simulink model "FD_example_2018b"  (R2018b)
settings: Solver=ode1  StartTime=0.0  StopTime=inf  FixedStep=1e-3  RelTol=1e-3
InitFcn:
  | plant = Dexmart_index;
  | plant_mdh = mdh_struct_to_matrix(plant.mdh_ori,1);
  | 
  | % init value for solver
  | q_init = zeros(plant.nj,1);
  | qD_init = zeros(plant.nj,1);
  | 
  | % parameters for passive properties
  | K_q = 1e1;% stiffness Nm/rad
  | q0_stiff = [0;pi/6;pi/4;pi/6];
  | D_q = 5; % Damping of joint
  | 
  | % parameter for controller
  | grv_comp_on = 0;
  | K_ctrl = 0;
  | D_ctrl = 0;
  | 
  | 
  | % desired x
  | 
  | x_desired = [rand(plant.nj,1);zeros(plant.nj,1)];
model workspace: external: MAT-File D:\repos\hand_modeling_toolbox\examples\hand_one\hand_one_model.mat (data not in the file)
values from neighbouring files (symbols this model uses):
  Dexmart_index = Finger('Index_Dexmart', 'type','R_RRRR', 'l_links',finger_index_dimension)    [create_Dexmart_index.m]
settings Model: Creator=ge26jow  LastModifiedBy=ge26jow
settings DataIOCC: ReturnWorkspaceOutputs=on
settings DebuggingCC: SFMachineParentedDataDiag=error

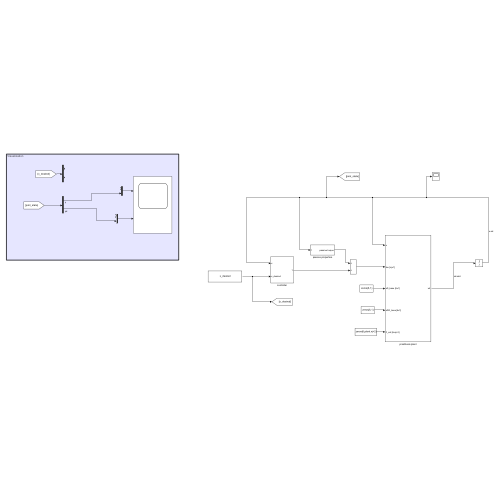
[thumbnail: Simulink's stored preview of the top-level diagram]
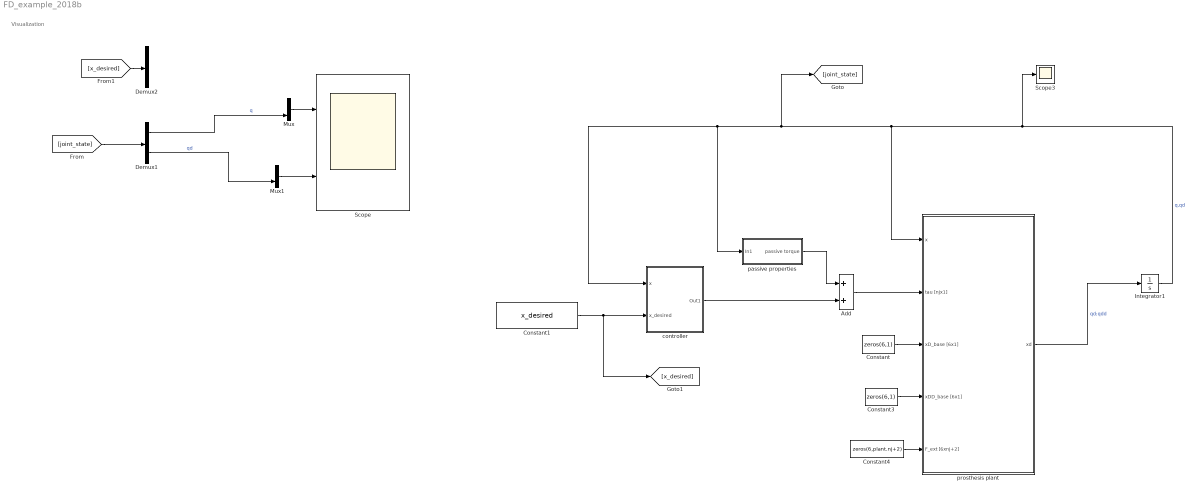
== system FD_example_2018b ==
  note: Visualization
  Add : Sum
  Constant : Constant  Value=zeros(6,1)
  Constant1 : Constant  Value=x_desired
  Constant3 : Constant  Value=zeros(6,1)
  Constant4 : Constant  Value=zeros(6,plant.nj+2)
  Demux1 : Demux  Outputs=[plant.nj,plant.nj]
  Demux2 : Demux  Outputs=[plant.nj,plant.nj]
  Integrator1 : Integrator  InitialCondition=[q_init;qD_init]  WrappedStateUpperValue=[pi,pi,pi,pi,1e4,1e4,1e4,1e4]  WrappedStateLowerValue=-[pi,pi,pi,pi,1e4,1e4,1e4,1e4]
  Mux : Mux  Inputs=2
  Mux1 : Mux  Inputs=2
  Scope : Scope  NumInputPorts=2
  Scope3 : Scope
  controller : Subsystem
  passive properties : Subsystem
  prosthesis plant : Subsystem
  wires:
  Add/1 -> prosthesis plant/2(tau [njx1])
  prosthesis plant/1(xd) -> Integrator1/1  "qd;qdd"
  Integrator1/1 -> [joint_state], controller/1(x), passive properties/1(In1), prosthesis plant/1(x), Scope3/1  "q,qd"
  Constant/1 -> prosthesis plant/3(xD_base [6x1])
  Constant3/1 -> prosthesis plant/4(xDD_base [6x1])
  Constant4/1 -> prosthesis plant/5(F_ext [6xnj+2])
  passive properties/1(passive torque) -> Add/1
  [joint_state] -> Demux1/1
  controller/1(Out1) -> Add/2
  Constant1/1 -> [x_desired], controller/2(x_desired)
  [x_desired] -> Demux2/1
  Demux1/1 -> Mux/2  "q"
  Mux/1 -> Scope/1
  Mux1/1 -> Scope/2
  Demux1/2 -> Mux1/2  "qd"

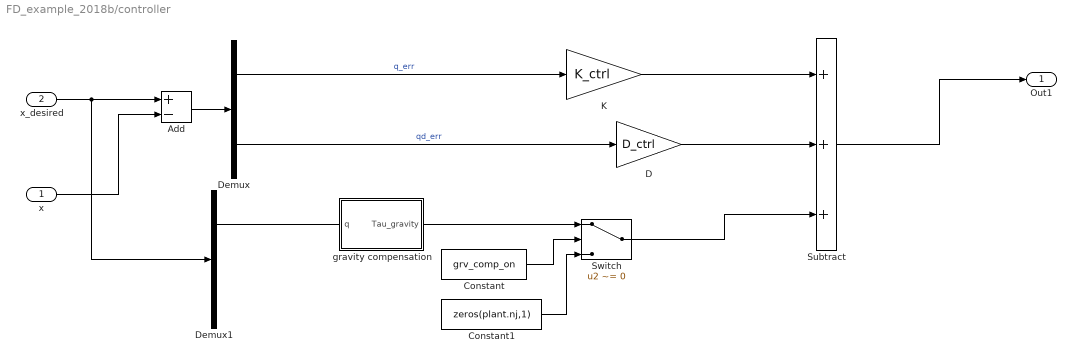
== system FD_example_2018b/controller ==
  x : Inport
  x_desired : Inport  Port=2
  Add : Sum  Inputs=+-
  Constant : Constant  Value=grv_comp_on
  Constant1 : Constant  Value=zeros(plant.nj,1)
  D : Gain  Gain=D_ctrl
  Demux : Demux  Outputs=[plant.nj,plant.nj]
  Demux1 : Demux  Outputs=[plant.nj,plant.nj]
  K : Gain  Gain=K_ctrl
  Subtract : Sum  Inputs=+++
  Switch : Switch  Criteria=u2 ~= 0
  gravity compensation : Subsystem
  Out1 : Outport
  wires:
  K/1 -> Subtract/1
  D/1 -> Subtract/2
  Subtract/1 -> Out1/1
  Demux/2 -> D/1  "qd_err"
  Demux/1 -> K/1  "q_err"
  Add/1 -> Demux/1
  x/1 -> Add/2
  x_desired/1 -> Demux1/1, Add/1
  Demux1/1 -> gravity compensation/1(q)
  Constant/1 -> Switch/2
  gravity compensation/1(Tau_gravity) -> Switch/1
  Switch/1 -> Subtract/3
  Constant1/1 -> Switch/3

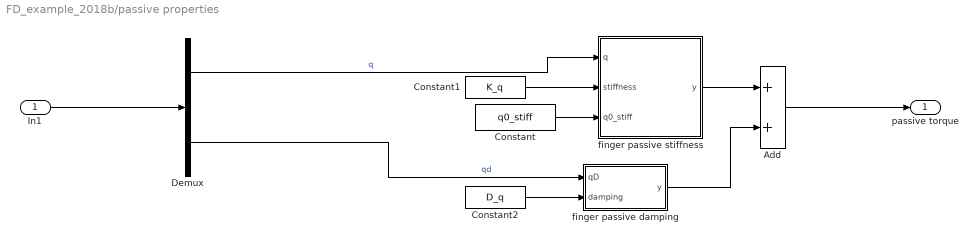
== system FD_example_2018b/passive properties ==
  In1 : Inport
  Add : Sum
  Constant : Constant  Value=q0_stiff
  Constant1 : Constant  Value=K_q
  Constant2 : Constant  Value=D_q
  Demux : Demux  Outputs=[plant.nj,plant.nj]
  finger passive damping : MATLAB Function  TreatAsAtomicUnit=on
  finger passive stiffness : MATLAB Function  TreatAsAtomicUnit=on
  passive torque : Outport
  wires:
  Constant2/1 -> finger passive damping/2(damping)
  finger passive damping/1(y) -> Add/2
  Demux/2 -> finger passive damping/1(qD)  "qd"
  Constant1/1 -> finger passive stiffness/2(stiffness)
  finger passive stiffness/1(y) -> Add/1
  Demux/1 -> finger passive stiffness/1(q)  "q"
  In1/1 -> Demux/1
  Constant/1 -> finger passive stiffness/3(q0_stiff)
  Add/1 -> passive torque/1

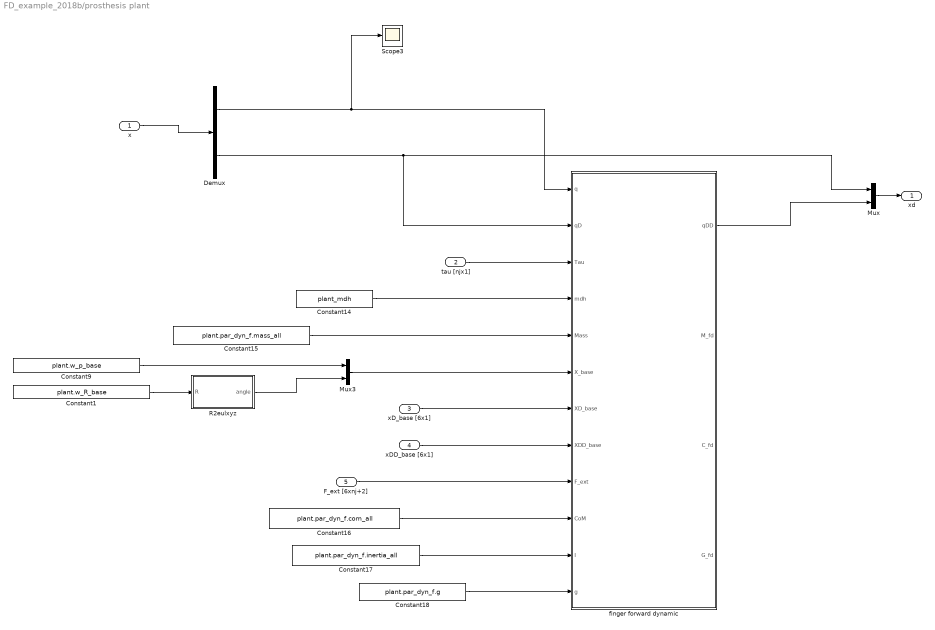
== system FD_example_2018b/prosthesis plant ==
  x : Inport
  tau [njx1] : Inport  Port=2
  xD_base [6x1] : Inport  Port=3
  xDD_base [6x1] : Inport  Port=4
  F_ext [6xnj+2] : Inport  Port=5
  Constant1 : Constant  Value=plant.w_R_base
  Constant14 : Constant  Value=plant_mdh
  Constant15 : Constant  Value=plant.par_dyn_f.mass_all
  Constant16 : Constant  Value=plant.par_dyn_f.com_all
  Constant17 : Constant  Value=plant.par_dyn_f.inertia_all
  Constant18 : Constant  Value=plant.par_dyn_f.g
  Constant9 : Constant  Value=plant.w_p_base
  Demux : Demux  Outputs=[plant.nj,plant.nj]
  Mux : Mux  Inputs=2
  Mux3 : Mux  Inputs=[3,3]
  R2eulxyz : MATLAB Function  TreatAsAtomicUnit=on
  Scope3 : Scope
  finger forward dynamic : MATLAB Function  TreatAsAtomicUnit=on
  xd : Outport
  wires:
  Constant18/1 -> finger forward dynamic/12(g)
  tau [njx1]/1 -> finger forward dynamic/3(Tau)
  Constant17/1 -> finger forward dynamic/11(I)
  finger forward dynamic/1(qDD) -> Mux/2
  Demux/2 -> finger forward dynamic/2(qD), Mux/1
  Mux3/1 -> finger forward dynamic/6(X_base)
  Constant14/1 -> finger forward dynamic/4(mdh)
  Demux/1 -> Scope3/1, finger forward dynamic/1(q)
  F_ext [6xnj+2]/1 -> finger forward dynamic/9(F_ext)
  Constant15/1 -> finger forward dynamic/5(Mass)
  Constant16/1 -> finger forward dynamic/10(CoM)
  Mux/1 -> xd/1
  Constant1/1 -> R2eulxyz/1(R)
  R2eulxyz/1(angle) -> Mux3/2
  Constant9/1 -> Mux3/1
  x/1 -> Demux/1
  xD_base [6x1]/1 -> finger forward dynamic/7(XD_base)
  xDD_base [6x1]/1 -> finger forward dynamic/8(XDD_base)

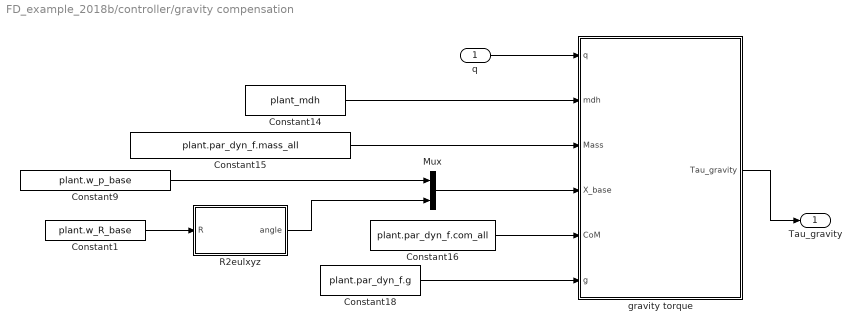
== system FD_example_2018b/controller/gravity compensation ==
  q : Inport
  Constant1 : Constant  Value=plant.w_R_base
  Constant14 : Constant  Value=plant_mdh
  Constant15 : Constant  Value=plant.par_dyn_f.mass_all
  Constant16 : Constant  Value=plant.par_dyn_f.com_all
  Constant18 : Constant  Value=plant.par_dyn_f.g
  Constant9 : Constant  Value=plant.w_p_base
  Mux : Mux  Inputs=[3,3]
  R2eulxyz : MATLAB Function  TreatAsAtomicUnit=on
  "gravity torque " : MATLAB Function  TreatAsAtomicUnit=on
  Tau_gravity : Outport
  wires:
  Constant14/1 -> "gravity torque "/2(mdh)
  Constant16/1 -> "gravity torque "/5(CoM)
  Mux/1 -> "gravity torque "/4(X_base)
  Constant18/1 -> "gravity torque "/6(g)
  Constant15/1 -> "gravity torque "/3(Mass)
  "gravity torque "/1(Tau_gravity) -> Tau_gravity/1
  q/1 -> "gravity torque "/1(q)
  Constant1/1 -> R2eulxyz/1(R)
  Constant9/1 -> Mux/1
  R2eulxyz/1(angle) -> Mux/2

== matlab function FD_example_2018b/prosthesis plant/finger forward dynamic ==
  data: q input; qDD output; qD input; Tau input; mdh input; Mass input; X_base input; XD_base input; XDD_base input; F_ext input; CoM input; I input; g input; M_fd output; C_fd output; G_fd output
% recursive Newton-Euler method to compute inverse dynamic with mdh
% parameters
% Input:
%     q,qD:             [n_qx1] joint states
%     Tau               [n_q] joint torque
%     mdh:              [n_q+1x4] in sequence of [alpha,a,theta,d] To be
%                       noted that the theta should exclude from mdh parameters 
%     Mass:             [n_q+1] mass vector. the first mass is the base 
%     X_base:           [6x1] eulerxyz
%     XD_base:          [6x1] translational and angular velocity
%     F_ext:            [6x1] force/moment that exerted by the environment to the endeffector frame. 
%     CoM:              [3xn_q+1] in local frame; last column is endeffector
%     I:                [6xn_q+1] in local frame with respect to center of mass. in sequence of [xx yy zz yz xz xy]
%     g:                [3x1] gravity term
% 
% Output:
%     qDD:              [n_qx1] joint acceleration 
%     M_fd:             [n_qxn_q] Mass matrix 
%     C_fd:             [n_q] velocity-dependent torque 
%     G_fd:             [n_q] gravity torque  

function [qDD,M_fd,C_fd,G_fd] = fordyn_ne_mdh(q,qD,Tau,mdh, Mass, X_base, XD_base,XDD_base, F_ext, CoM, I, g)
coder.extrinsic('invdyn_ne_mdh_mex');

n_q = length(q);
% assert(n_q == length(qD)&&n_q == length(Tau),'fordyn_ne_mdh: dimension error!');

mex = 1;


M_fd = zeros(n_q,n_q);
G_fd = zeros(n_q,1);
C_fd = zeros(n_q,1);

% gravity term
if mex
    G_fd = invdyn_ne_mdh_mex(q,zeros(n_q,1),zeros(n_q,1),mdh, Mass,...
        X_base, XD_base, XDD_base, zeros(6,1), CoM, I, g);
else
    G_fd = invdyn_ne_mdh(q,zeros(n_q,1),zeros(n_q,1),mdh, Mass,...
        X_base, XD_base, XDD_base, zeros(6,1), CoM, I, g);
end
% C term
if mex
    C_fd = invdyn_ne_mdh_mex(q,qD,zeros(n_q,1),mdh, Mass,...
        X_base, XD_base, XDD_base, zeros(6,1), CoM, I, g);
else
    C_fd = invdyn_ne_mdh(q,qD,zeros(n_q,1),mdh, Mass,...
             X_base, XD_base, XDD_base, zeros(6,1), CoM, I, g);
end
C_fd = C_fd - G_fd;

% M term
M_fd = zeros(n_q,n_q);

for i = 1:n_q
    qDD_M = zeros(n_q,1);
    qDD_M(i) = 1;
    if mex
        M_fd(:,i) = invdyn_ne_mdh_mex(q,zeros(n_q,1),qDD_M,mdh, Mass,...
            X_base, XD_base, XDD_base, zeros(6,1), CoM, I, g);
    else
        M_fd(:,i) = invdyn_ne_mdh(q,zeros(n_q,1),qDD_M,mdh, Mass,...
            X_base, XD_base, XDD_base, zeros(6,1), CoM, I, g);
    end
    M_fd(:,i) = M_fd(:,i) - G_fd;
end

% use Jacobian_geom_mdh.m to calculate geometric Jacobian
w_R_b = euler2R_XYZ(X_base(4:6));
b_J = Jacobian_geom_mdh(mdh,q);
J_ne = blkdiag(w_R_b,w_R_b)*b_J;
tau_ext = zeros(n_q,1);
for i = 1:n_q+1
    mdh_i = mdh(1:i,:);
    q_i = q(1:min(i,n_q));
    b_J_i = zeros(6,n_q);
    b_J_i(:,1:min(i,n_q)) =  Jacobian_geom_mdh(mdh_i,q_i);
    J_ne_i= blkdiag(w_R_b,w_R_b)*b_J_i;
    tau_i = J_ne_i'*F_ext(:,i+1);
    tau_ext = tau_ext + tau_i;
end


qDD = (M_fd)\(Tau + tau_ext - G_fd - C_fd);


end

== matlab function FD_example_2018b/passive properties/finger passive stiffness ==
  data: q input; y output; stiffness input; q0_stiff input
function y = fcn(q,stiffness,q0_stiff)

y = -stiffness.*(q-q0_stiff);

== matlab function FD_example_2018b/passive properties/finger passive damping ==
  data: qD input; y output; damping input
function y = fcn(qD,damping)

y = -damping.*qD;

== matlab function FD_example_2018b/controller/gravity compensation/gravity torque  ==
  data: q input; Tau_gravity output; mdh input; Mass input; X_base input; CoM input; g input
function Tau_gravity = fcn(q,mdh, Mass, X_base, CoM, g)

Tau_gravity = invdyn_ne_mdh_all_fext_gravity(q,mdh, Mass, X_base, CoM, g);

== matlab function FD_example_2018b/controller/gravity compensation/R2eulxyz ==
  data: R input; angle output
function angle = fcn(R)

angle = R2euler_XYZ(R);

== matlab function FD_example_2018b/prosthesis plant/R2eulxyz ==
  data: R input; angle output
function angle = fcn(R)

angle = R2euler_XYZ(R);
